simulink model "sampleModel71"  (R2021a)
settings: Solver=VariableStepAuto  StartTime=0.0  StopTime=10.0  RelTol=1e-3
undefined symbols (not defined in the file): Newton, Raphson
libraries: simulink x6
settings Model: Creator=user  LastModifiedBy=user

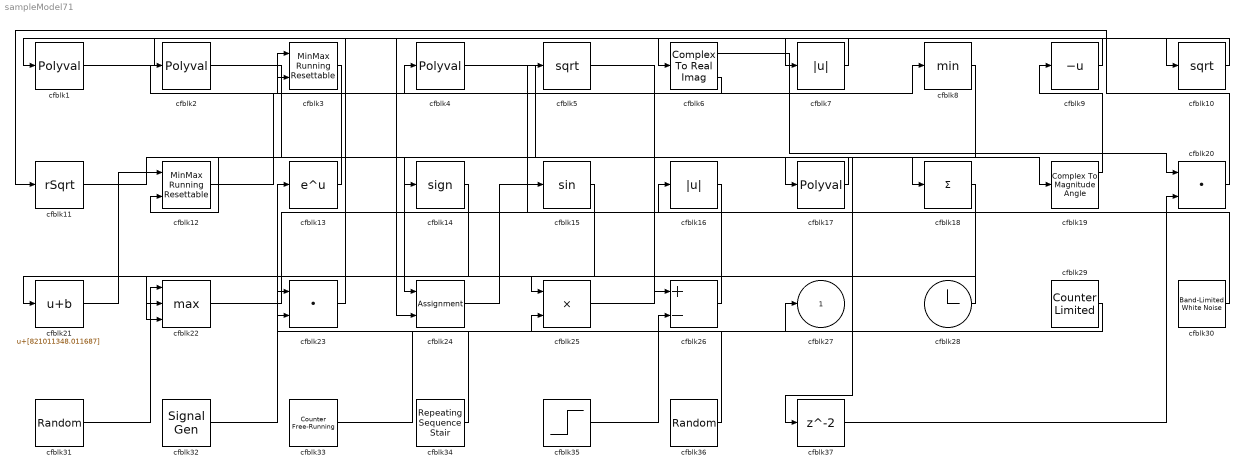
== system sampleModel71 ==
  cfblk{1..2,4,17} (4 alike) : Polyval  Coefs=[ +2.081618890e-019, -1.441693666e-014, +4.719686976e-010, -8.536869453e-006, +1.621573104e-001, -8.087801117e+001 ]
  cfblk10 : Sqrt  SaturateOnIntegerOverflow=on
  cfblk11 : Sqrt  Operator=rSqrt  AlgorithmType=Newton-Raphson  SaturateOnIntegerOverflow=on
  cfblk12 : simulink/Math Operations/MinMax Running Resettable  Function=min  vinit=0.0
  cfblk13 : Math  SaturateOnIntegerOverflow=on
  cfblk14 : Signum
  cfblk15 : Trigonometry
  cfblk16 : Abs
  cfblk18 : Sum  Inputs=+
  cfblk19 : ComplexToMagnitudeAngle
  cfblk20 : DotProduct  InputSameDT=on  OutDataTypeStr=Inherit: Inherit via internal rule
  cfblk21 : Bias  Bias=[821011348.011687]
  cfblk22 : MinMax  Function=max  Inputs=3
  cfblk23 : DotProduct  InputSameDT=on  OutDataTypeStr=Inherit: Inherit via internal rule
  cfblk24 : Assignment  DiagnosticForDimensions=Warning  IndexOptions=Index vector (dialog)  Indices=1  OutputSizes=1
  cfblk25 : Product  Inputs=**
  cfblk26 : Sum  Inputs=+-
  cfblk28 : Clock
  cfblk29 : simulink/Sources/Counter Limited  uplimit=[90.000000]  tsamp=-1
  cfblk3 : simulink/Math Operations/MinMax Running Resettable  Function=min  vinit=0.0
  cfblk30 : simulink/Sources/Band-Limited White Noise  Cov=[9683588534.844969]  Ts=0.1  seed=[6647796679.000000]
  cfblk31 : RandomNumber  Mean=[-77362.465379]  Variance=[8276.617076]  Seed=[35855637.000000]  SampleTime=0.1
  cfblk32 : SignalGenerator  WaveForm=sawtooth  Amplitude=[143946783.164193]
  cfblk33 : simulink/Sources/Counter Free-Running  NumBits=[59.000000]  tsamp=-1
  cfblk34 : simulink/Sources/Repeating Sequence Stair  OutValues=[210212115.474724, -265525901.278402]  tsamp=-1  OutMin=[]  OutMax=[]  OutDataTypeStr=double  OutputDataTypeScalingMode=double  OutDataType=fixdt(0,8)  ConRadixGroup=Best Precision: Vector-wise  OutScaling=2^-12
  cfblk35 : Step  Time=[1.000000]  Before=[-529109176.246903]  After=[358542803.470678]  SampleTime=0
  cfblk36 : UniformRandomNumber  Minimum=[-5709913592.057831]  Maximum=[1662818118.310796]  Seed=[54274275.000000]  SampleTime=0.1
  cfblk37 : Delay  SampleTime=1
  cfblk5 : Sqrt  SaturateOnIntegerOverflow=on
  cfblk6 : ComplexToRealImag
  cfblk7 : Abs
  cfblk8 : MinMax
  cfblk9 : UnaryMinus
  cfblk27 : Outport
  wires:
  cfblk30/1 -> cfblk16/1
  cfblk34/1 -> cfblk13/1
  cfblk17/1 -> cfblk24/1
  cfblk24/1 -> cfblk15/1
  cfblk6/1 -> cfblk20/1
  cfblk21/1 -> cfblk12/1
  cfblk5/1 -> cfblk26/1
  cfblk9/1 -> cfblk24/2
  cfblk4/1 -> cfblk17/1
  cfblk3/1 -> cfblk12/2
  cfblk25/1 -> cfblk8/1
  cfblk23/1 -> cfblk1/1
  cfblk15/1 -> cfblk25/1
  cfblk29/1 -> cfblk25/2
  cfblk20/1 -> cfblk11/1
  cfblk1/1 -> cfblk10/1
  cfblk2/1 -> cfblk19/1
  cfblk11/1 -> cfblk18/1
  cfblk19/1 -> cfblk9/1
  cfblk31/1 -> cfblk22/1
  cfblk16/1 -> cfblk22/2
  cfblk22/1 -> cfblk5/1
  cfblk35/1 -> cfblk26/2
  cfblk18/1 -> cfblk21/1
  cfblk10/1 -> cfblk7/1
  cfblk26/1 -> cfblk3/1
  cfblk28/1 -> cfblk14/1
  cfblk6/2 -> cfblk2/1
  cfblk14/1 -> cfblk22/3
  cfblk7/1 -> cfblk6/1
  cfblk12/1 -> cfblk4/1
  cfblk33/1 -> cfblk27/1
  cfblk13/1 -> cfblk3/2
  cfblk36/1 -> cfblk23/1
  cfblk32/1 -> cfblk23/2
  cfblk8/1 -> cfblk37/1
  cfblk37/1 -> cfblk20/2
